simulink model "Stabi_Simu"  (R2022b)
settings: Solver=FixedStepAuto  StartTime=0.0  StopTime=1  FixedStep=0.0001  RelTol=1e-3
model workspace (MAT data in the model file):
  D = 0.06336
  I = 0.340909090909
  J = 0.0025
  P = 0.3
  g = 9.81
  l = 0.08
  m = 0.6
  phi_start = 0.174532925199
libraries: slpidlib x1
settings Model: Creator=Fabius  LastModifiedBy=Fabius

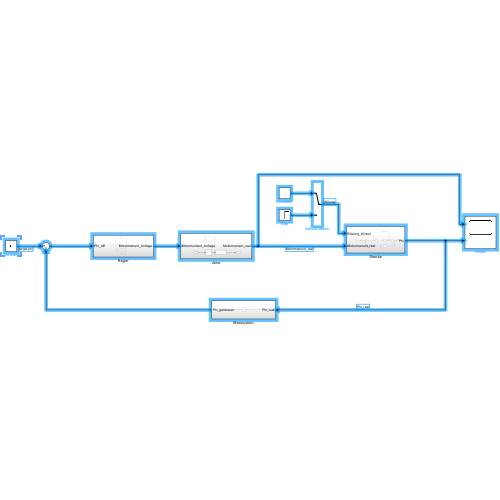
[thumbnail: Simulink's stored preview of the top-level diagram]
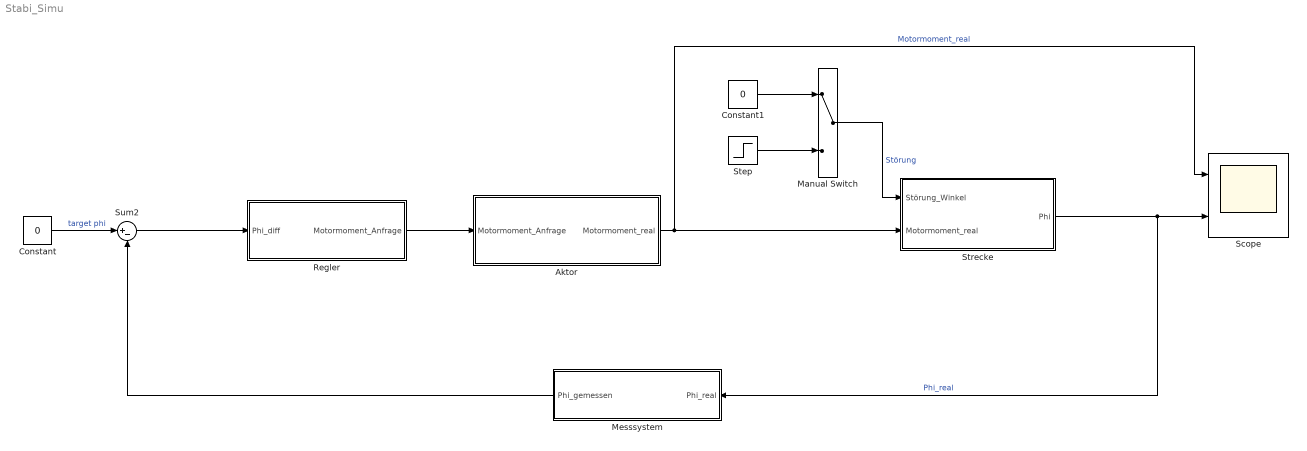
== system Stabi_Simu ==
  Aktor : Subsystem
  Constant : Constant  Value=0
  Constant1 : Constant  Value=0
  Manual Switch : ManualSwitch
  Messsystem : Subsystem
  Regler : Subsystem
  Scope : Scope  NumInputPorts=2
  Step : Step  After=10/360*2*pi  SampleTime=0
  Strecke : Subsystem
  Sum2 : Sum  Inputs=|+-
  wires:
  Step/1 -> Manual Switch/2
  Constant/1 -> Sum2/1  "target phi"
  Constant1/1 -> Manual Switch/1
  Messsystem/1(Phi_gemessen) -> Sum2/2
  Aktor/1(Motormoment_real) -> Strecke/2(Motormoment_real), Scope/1  "Motormoment_real"
  Sum2/1 -> Regler/1(Phi_diff)
  Regler/1(Motormoment_Anfrage) -> Aktor/1(Motormoment_Anfrage)
  Strecke/1(Phi) -> Messsystem/1(Phi_real), Scope/2  "Phi_real"
  Manual Switch/1 -> Strecke/1(Störung_Winkel)  "Störung"

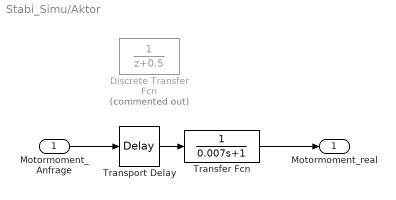
== system Stabi_Simu/Aktor ==
  Motormoment_Anfrage : Inport
  Discrete Transfer Fcn : DiscreteTransferFcn  Commented=on
  Transfer Fcn : TransferFcn  Denominator=[0.007 1]
  Transport Delay : TransportDelay  DelayTime=0.003
  Motormoment_real : Outport
  wires:
  Motormoment_Anfrage/1 -> Transport Delay/1
  Transport Delay/1 -> Transfer Fcn/1
  Transfer Fcn/1 -> Motormoment_real/1

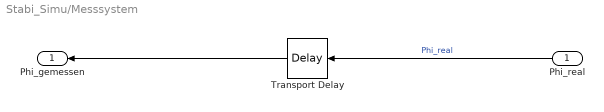
== system Stabi_Simu/Messsystem ==
  Phi_real : Inport
  Transport Delay : TransportDelay  DelayTime=0.003
  Phi_gemessen : Outport
  wires:
  Transport Delay/1 -> Phi_gemessen/1
  Phi_real/1 -> Transport Delay/1  "Phi_real"

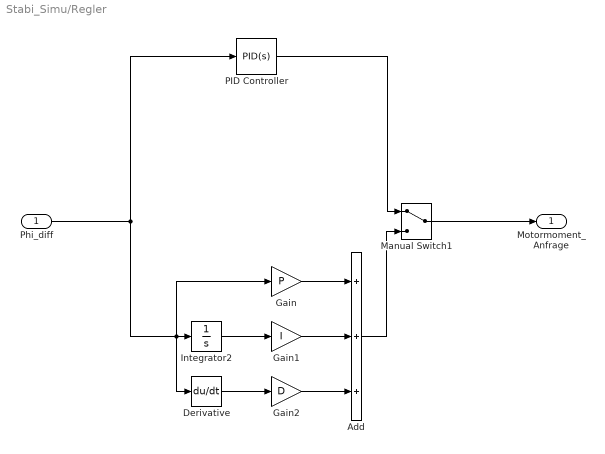
== system Stabi_Simu/Regler ==
  Phi_diff : Inport
  Add : Sum  Inputs=+++
  Derivative : Derivative
  Gain : Gain  Gain=P
  Gain1 : Gain  Gain=I
  Gain2 : Gain  Gain=D
  Integrator2 : Integrator
  Manual Switch1 : ManualSwitch
  PID Controller : slpidlib/PID Controller  Controller=PID  Form=Parallel  TimeDomain=Continuous-time  UseExternalTs=off  SampleTime=-1  IntegratorMethod=Forward Euler  FilterMethod=Forward Euler  ControllerParametersSource=internal  P=0.93869378978087  I=2.39876538859644  UseKiTs=off  D=0.0905271819516453  N=3589.05718033537  UseFilter=on  TunerSelectOption=Transfer Function Based (PID Tuner App)  InitialConditionSource=internal  InitialConditionForIntegrator=0  InitialConditionForFilter=0  DifferentiatorICPrevScaledInput=0  ExternalReset=none  TrackingMode=off  Kt=1  LimitOutput=off  SatLimitsSource=internal  UpperSaturationLimit=inf  LowerSaturationLimit=-inf  LinearizeAsGain=on  AntiWindupMode=none  Kb=1  LimitIntegrator=off  UpperIntegratorSaturationLimit=inf  LowerIntegratorSaturationLimit=-inf  POutMin=[]  POutMax=[]  IOutMin=[]  IOutMax=[]  DOutMin=[]  DOutMax=[]  NOutMin=[]  NOutMax=[]  SumOutMin=[]  SumOutMax=[]  SaturationOutMin=[]  SaturationOutMax=[]  PParamMin=[]  PParamMax=[]  IParamMin=[]  IParamMax=[]  DParamMin=[]  DParamMax=[]  NParamMin=[]  NParamMax=[]  KbParamMin=[]  KbParamMax=[]  KtParamMin=[]  KtParamMax=[]  KbOutMin=[]  KbOutMax=[]  KtOutMin=[]  KtOutMax=[]  IntegratorOutMin=[]  IntegratorOutMax=[]  FilterOutMin=[]  FilterOutMax=[]  SumI1OutMin=[]  SumI1OutMax=[]  SumI2OutMin=[]  SumI2OutMax=[]  SumI3OutMin=[]  SumI3OutMax=[]  SumI4OutMin=[]  SumI4OutMax=[]  SumDOutMin=[]  SumDOutMax=[]  DifferentiatorOutMin=[]  DifferentiatorOutMax=[]  FilterDiffOutCoefMin=[]  FilterDiffOutCoefMax=[]  ReciprocalOutMin=[]  ReciprocalOutMax=[]  SumDenOutMin=[]  SumDenOutMax=[]  SumNumOutMin=[]  SumNumOutMax=[]  DivideOutMin=[]  DivideOutMax=[]  UdiffTsProdOutMin=[]  UdiffTsProdOutMax=[]  NTsProdOutMin=[]  NTsProdOutMax=[]  UintegralTsProdOutMin=[]  UintegralTsProdOutMax=[]  UngainTsProdOutMin=[]  UngainTsProdOutMax=[]  ClampingZeroOutDataTypeStr=Inherit: Inherit via back propagation  ClampingZeroOutMin=[]  ClampingZeroOutMax=[]  FilterDenConstantOutDataTypeStr=Inherit: Inherit via back propagation  FilterDenConstantOutMin=[]  FilterDenConstantOutMax=[]  PCopyOutDataTypeStr=Inherit: Inherit via back propagation  PCopyOutMin=[]  PCopyOutMax=[]  NCopyOutDataTypeStr=Inherit: Inherit via back propagation  NCopyOutMin=[]  NCopyOutMax=[]  IntegratorContinuousStateAttributes=''  IntegratorStateMustResolveToSignalObject=off  IntegratorRTWStateStorageClass=Auto  FilterContinuousStateAttributes=''  FilterStateMustResolveToSignalObject=off  FilterRTWStateStorageClass=Auto  ParallelPVariant=InternalParameters  IdealPVariant=Disabled  IVariant=InternalParameters  DVariant=InternalParameters  IntegratorVariant=Continuous  SatVariant=Disabled  AWVariant=Passthrough  PCopyVariant=Disabled  TRVariant=Disabled  FdbkBlocksVariant=Forward  IdealPFdbkVariant=Disabled  SatFdbkVariant=Disabled  DerivativeFilterVariant=ContFilter  NVariant=InternalParameters  NCopyVariant=Disabled  FilterICVariant=InternalICsFilter  IntegratorICVariant=InternalICs  ExternalResetVariant=Disabled  TRSumVariant=Passthrough  SumFdbkVariant=Disabled  SumVariant=Sum_PID  TsampFilterVariant=InternalTs  TsampNgainVariant=Passthrough  TsampIntegralVariant=Passthrough  ExternalSaturationOutDataTypeStr=Inherit: Same as second input
  Motormoment_Anfrage : Outport
  wires:
  Phi_diff/1 -> Gain/1, Derivative/1, Integrator2/1, PID Controller/1
  PID Controller/1 -> Manual Switch1/1
  Add/1 -> Manual Switch1/2
  Integrator2/1 -> Gain1/1
  Derivative/1 -> Gain2/1
  Gain1/1 -> Add/2
  Manual Switch1/1 -> Motormoment_Anfrage/1
  Gain2/1 -> Add/3
  Gain/1 -> Add/1

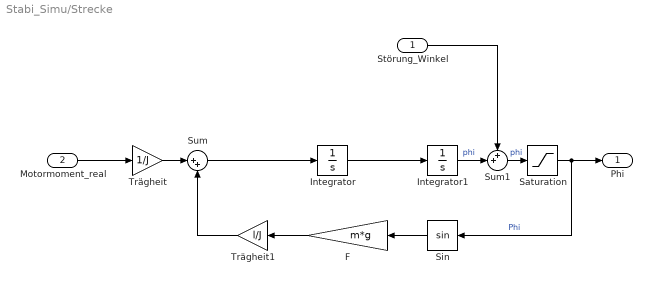
== system Stabi_Simu/Strecke ==
  Störung_Winkel : Inport
  Motormoment_real : Inport  Port=2
  F : Gain  Gain=m*g
  Integrator : Integrator
  Integrator1 : Integrator  InitialCondition=phi_start
  Saturation : Saturate  UpperLimit=pi/2  LowerLimit=-pi/2
  Sin : Trigonometry
  Sum : Sum  Inputs=|++
  Sum1 : Sum  Inputs=++|
  Trägheit : Gain  Gain=1/J
  Trägheit1 : Gain  Gain=l/J
  Phi : Outport
  wires:
  Motormoment_real/1 -> Trägheit/1
  Saturation/1 -> Phi/1, Sin/1  "Phi"
  Trägheit1/1 -> Sum/2
  Sum/1 -> Integrator/1
  Integrator1/1 -> Sum1/2  "phi"
  F/1 -> Trägheit1/1
  Sin/1 -> F/1
  Trägheit/1 -> Sum/1
  Sum1/1 -> Saturation/1  "phi"
  Integrator/1 -> Integrator1/1
  Störung_Winkel/1 -> Sum1/1
